simulink model "sim12ex9"  (Simulink 2.09)
settings: Solver=ode23  StartTime=0.0  StopTime=15  MaxStep=.05  RelTol=1e-3  AbsTol=1e-3
settings Model: SaveTime=off  SaveOutput=off  ConsistencyChecking=off  RTWTemplateMakefile=grt_vc.tmf

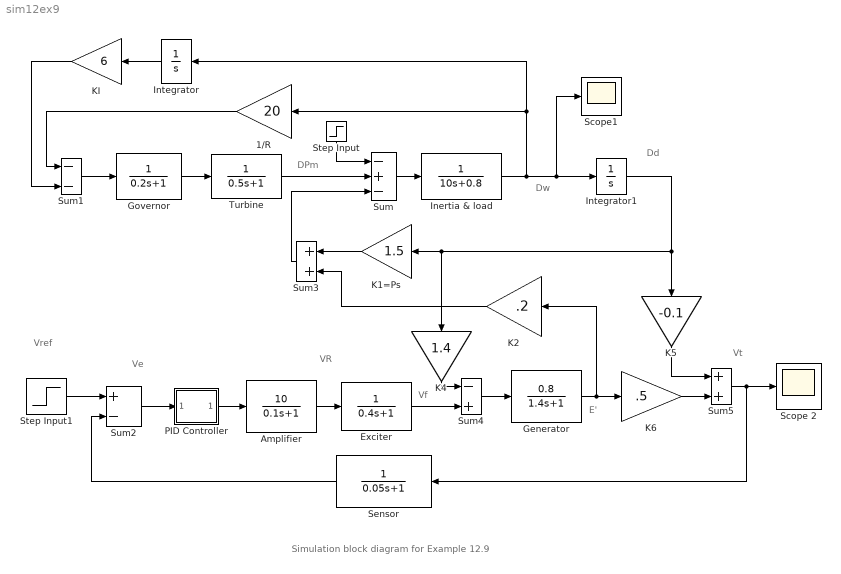
== system sim12ex9 ==
  note: Simulation block diagram for Example 12.9
  note: Dw
  note: Dd
  note: Vf
  note: VR
  note: E'
  note: Vt
  note: Ve
  note: Vref
  note: DPm
  1/R : Gain  Orientation=left  Gain=20
  Amplifier : TransferFcn  Numerator=10  Denominator="[0.1  1]"
  Exciter : TransferFcn  Numerator=1  Denominator="[0.4  1]"
  Generator : TransferFcn  Numerator=[0.8]  Denominator=[ 1.4 1]
  Governor : TransferFcn  Numerator=[1]  Denominator="[0.2   1]"
  Inertia & load : TransferFcn  Numerator=[1]  Denominator="[10  0.8]"
  Integrator : Integrator  Orientation=left  ExternalReset=none  InitialConditionSource=internal  InitialCondition=0  LimitOutput=off  UpperSaturationLimit=inf  LowerSaturationLimit=-inf  ShowSaturationPort=off  ShowStatePort=off  AbsoluteTolerance=auto
  Integrator1 : Integrator  ExternalReset=none  InitialConditionSource=internal  InitialCondition=0  LimitOutput=off  UpperSaturationLimit=inf  LowerSaturationLimit=-inf  ShowSaturationPort=off  ShowStatePort=off  AbsoluteTolerance=auto
  K1=Ps : Gain  Orientation=left  Gain=1.5
  K2 : Gain  Orientation=left  Gain=.2
  K4 : Gain  Orientation=down  Gain=1.4
  K5 : Gain  Orientation=down  Gain=-0.1
  K6 : Gain  Gain=.5
  KI : Gain  Orientation=left  Gain=6
  PID Controller : Subsystem  mask(PID Controller){@1=1, @2=0.25, @3=0.3}
      mask prompts: @1 "Proportional:"; @2 "Integral"; @3 "Derivative:"
      mask help:
      | Enter expressions for proportional, integral, and derivative terms.
      | P+I/s+Ds
      mask init:
      | P=@1; I=@2; D=@3;
      mask Help: This block implements a PID controller where parameters are entered for the Proportional, Integral and Derivative terms. Unmask this block to see how it works. The derivative term is implemented using a true derivative block.
      mask Display: disp('PID')
  Scope 2 : Scope
      settings: TickLabels=on  TimeRange=auto  YMin=-5  YMax=5  SaveToWorkspace=off  SaveName=ScopeData
  Scope1 : Scope
      settings: TickLabels=on  TimeRange=auto  YMin=-5  YMax=5  SaveToWorkspace=off  SaveName=ScopeData
  Sensor : TransferFcn  Orientation=left  Numerator=[1]  Denominator="[0.05  1]"
  Step Input : Step  Orientation=down  Time=2  Before=0.2  After=.2
  Step Input1 : Step  Time=12  Before=1  After=1
  Sum : Sum  Inputs=-+-
  Sum1 : Sum  Inputs=--
  Sum2 : Sum  Inputs=+-
  Sum3 : Sum  Orientation=left  Inputs=++
  Sum4 : Sum  Inputs=-+
  Sum5 : Sum  Inputs=++
  Turbine : TransferFcn  Numerator=[1]  Denominator="[0.5  1]"
  wires:
  Inertia & load/1 -> 1/R/1, Integrator/1, Scope1/1, Integrator1/1
  Integrator1/1 -> K4/1, K1=Ps/1, K5/1
  KI/1 -> Sum1/2
  Integrator/1 -> KI/1
  1/R/1 -> Sum1/1
  K2/1 -> Sum3/2
  K4/1 -> Sum4/1
  Generator/1 -> K2/1, K6/1
  Sum5/1 -> Sensor/1, Scope 2/1
  K5/1 -> Sum5/1
  K1=Ps/1 -> Sum3/1
  K6/1 -> Sum5/2
  Sum4/1 -> Generator/1
  Exciter/1 -> Sum4/2
  Sum3/1 -> Sum/3
  PID Controller/1(Out_1) -> Amplifier/1
  Sum2/1 -> PID Controller/1(In_1)
  Amplifier/1 -> Exciter/1
  Sensor/1 -> Sum2/2
  Step Input1/1 -> Sum2/1
  Step Input/1 -> Sum/1
  Sum1/1 -> Governor/1
  Sum/1 -> Inertia & load/1
  Turbine/1 -> Sum/2
  Governor/1 -> Turbine/1

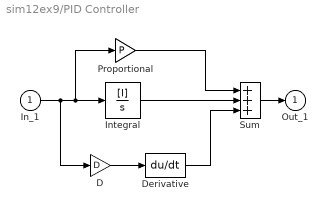
== system sim12ex9/PID Controller ==
  In_1 : Inport  Port=1  PortWidth=-1  SampleTime=-1
  D : Gain  Gain=D
  Derivative : Derivative
  Integral : TransferFcn  Numerator=[I]  Denominator=[1 0]
  Proportional : Gain  Gain=P
  Sum : Sum  Inputs=+++
  Out_1 : Outport  Port=1  InitialOutput=0
  wires:
  Proportional/1 -> Sum/1
  Integral/1 -> Sum/2
  Derivative/1 -> Sum/3
  In_1/1 -> Proportional/1, Integral/1, D/1
  Sum/1 -> Out_1/1
  D/1 -> Derivative/1
